simulink model "simulink_main"  (R2014b)
settings: Solver=ode45  StartTime=0.0  StopTime=3  RelTol=1e-3
values from neighbouring files (symbols this model uses):
  state_initial = [0 0 3 0 0 0 0 0 0 0 0 0]    [main.m]
settings Model: Creator=shuoli  LastModifiedBy=shuoli

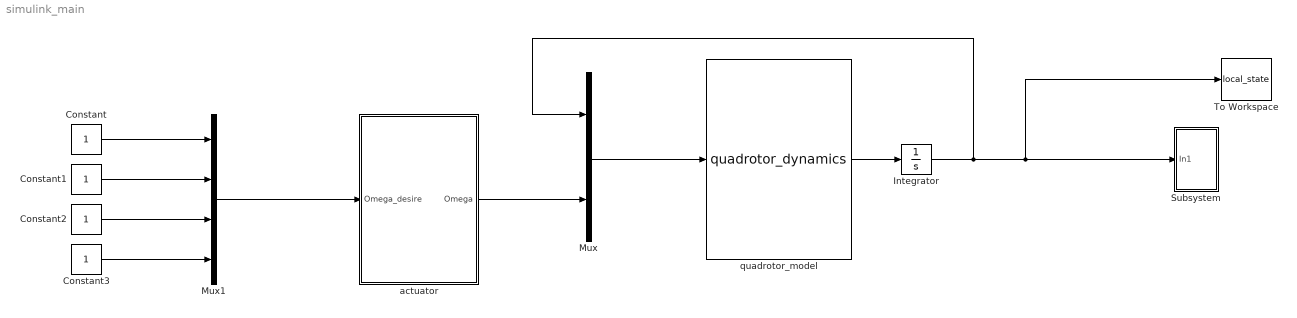
== system simulink_main ==
  Constant{,1..3} (4 alike) : Constant
  Integrator : Integrator  InitialCondition=state_initial
  Mux : Mux  Inputs=2
  Mux1 : Mux
  Subsystem : Subsystem
  To Workspace : ToWorkspace  VariableName=local_state  SampleTime=-1
      settings: Save2DSignal=2-D array (concatenate along first dimension)
  actuator : Subsystem
  quadrotor_model : MATLABFcn  MATLABFcn=quadrotor_dynamics
  wires:
  quadrotor_model/1 -> Integrator/1
  Mux/1 -> quadrotor_model/1
  Integrator/1 -> Mux/1, To Workspace/1, Subsystem/1(In1)
  actuator/1(Omega) -> Mux/2
  Mux1/1 -> actuator/1(Omega_desire)
  Constant/1 -> Mux1/1
  Constant1/1 -> Mux1/2
  Constant2/1 -> Mux1/3
  Constant3/1 -> Mux1/4

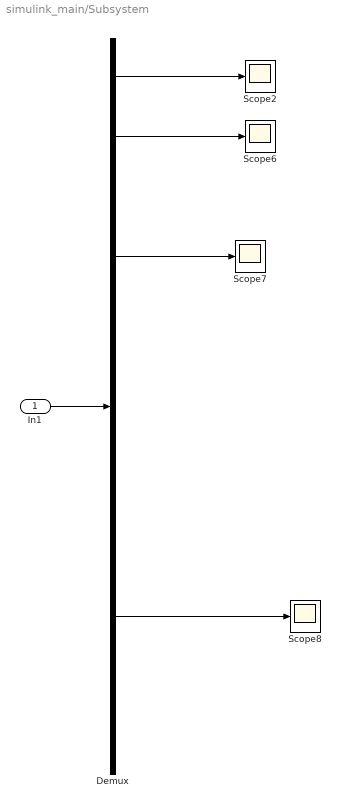
== system simulink_main/Subsystem ==
  In1 : Inport
  Demux : Demux  Outputs=12
  Scope{2,6..8} (4 alike) : Scope
      Scope2 settings: YMin=-18500  YMax=-16500  SaveName=ScopeData2
      Scope6 settings: YMax=2  SaveName=ScopeData6
      Scope7 settings: YMin=-4.3788e-74  YMax=0.2  SaveName=ScopeData7
      Scope8 settings: YMax=2  SaveName=ScopeData8
  wires:
  In1/1 -> Demux/1
  Demux/1 -> Scope2/1
  Demux/2 -> Scope6/1
  Demux/4 -> Scope7/1
  Demux/10 -> Scope8/1

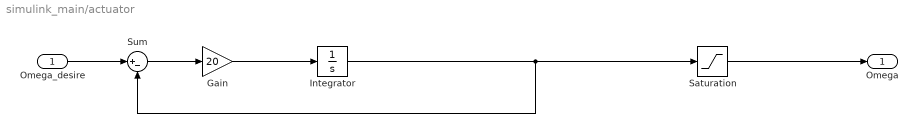
== system simulink_main/actuator ==
  Omega_desire : Inport
  Gain : Gain  Gain=20
  Integrator : Integrator  InitialCondition=[4477,4477,4477,4477]
  Saturation : Saturate  UpperLimit=10000  LowerLimit=0
  Sum : Sum  Inputs=|+-
  Omega : Outport
  wires:
  Integrator/1 -> Saturation/1, Sum/2
  Omega_desire/1 -> Sum/1
  Sum/1 -> Gain/1
  Gain/1 -> Integrator/1
  Saturation/1 -> Omega/1
